simulink model "freeze_cntr_blk"  (R2019a)
settings: Solver=VariableStepAuto  StartTime=0.0  StopTime=40  RelTol=1e-3
libraries: xbsIndex_r4 x2
settings Model: Creator=mybur  LastModifiedBy=mybur

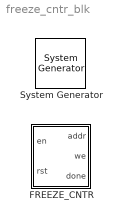
== system freeze_cntr_blk ==
  " System Generator" : xbsIndex_r4/ System Generator  Tag=genX  xilinxfamily=kintex7  part=xc7k325t  speed=-3  package=fbg676  synthesis_tool=Vivado  clock_wrapper=Clock Enables  directory=./netlist  proj_type=Vivado  Synth_file=Vivado Synthesis Defaults  Impl_file=Vivado Implementation Defaults  testbench=off  simulink_period=1  sysclk_period=10  dcm_input_clock_period=10  incr_netlist=off  trim_vbits=Everywhere in SubSystem  dbl_ovrd=According to Block Masks  core_generation=According to Block Masks  run_coregen=off  deprecated_control=off  eval_field=0  block_type=sysgen
  FREEZE_CNTR : Subsystem  mask(freeze_cntr){CounterBits=5}
      mask prompts: CounterBits "Counter Length (2^?)"
      mask help:
      | A freeze counter is an enabled counter which holds its final value (regardless of enables)
      | until it is reset.
      mask init:
      | Simulink.Block.eval([gcb, '/freeze_cntr']);

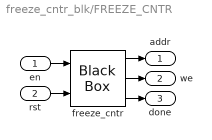
== system freeze_cntr_blk/FREEZE_CNTR ==
  en : Inport
  rst : Inport  Port=2
  freeze_cntr : xbsIndex_r4/Black Box  init_code=freeze_cntr_config  sim_method=ISE Simulator  verbose=off  block_type=blackbox2
  addr : Outport
  we : Outport  Port=2
  done : Outport  Port=3
  wires:
  en/1 -> freeze_cntr/1
  freeze_cntr/1 -> addr/1
  rst/1 -> freeze_cntr/2
  freeze_cntr/2 -> we/1
  freeze_cntr/3 -> done/1
